simulink model "scheme"  (R2024a)
settings: Solver=VariableStepAuto  StartTime=0.0  StopTime=100  RelTol=1e-3
InitFcn:
  | A=[1 0; 1 1];
  | b=[3; 5];
  | d=b;
  | 
  | A0f=[0 1; -16 -8];
  | b0f=[0; 1];
  | N=b0f/d;
  | 
  | Ad=[0 1; -10.24 -6.4];
  | H=[1 0];
  | M=lyap(A,-Ad,-b*H);
  | K=H*inv(M);
  | Am=A-b*K;
  | Q=eye(2);
  | P=lyap(Am',Q);
settings Model: Creator=User  LastModifiedBy=alexe

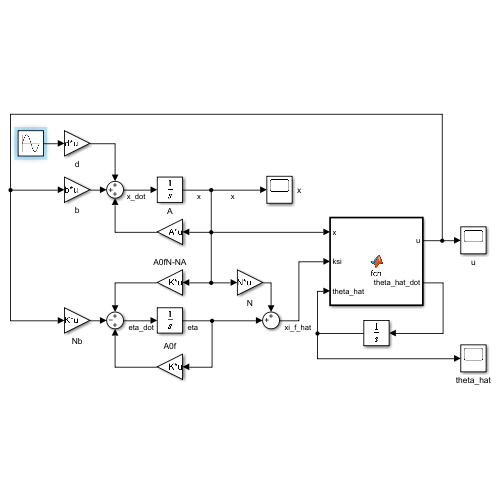
[thumbnail: Simulink's stored preview of the top-level diagram]
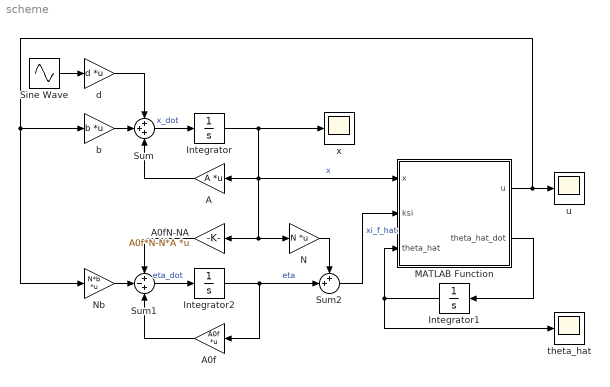
== system scheme ==
  A : Gain  Gain=A  Multiplication=Matrix(K*u)
  A0f : Gain  Gain=A0f  Multiplication=Matrix(K*u)
  A0fN-NA : Gain  Gain=A0f*N-N*A  Multiplication=Matrix(K*u)
  Integrator : Integrator  InitialCondition=[0; 0]
  Integrator1 : Integrator  InitialCondition=[0; 0]
  Integrator2 : Integrator  InitialCondition=[0; 0]
  MATLAB Function : MATLAB Function  TreatAsAtomicUnit=on
  N : Gain  Gain=N  Multiplication=Matrix(K*u)
  Nb : Gain  Gain=N*b  Multiplication=Matrix(K*u)
  Sine Wave : Sin  Amplitude=20  SampleTime=0
  Sum : Sum  Inputs=+++
  Sum1 : Sum  Inputs=+-+
  Sum2 : Sum  Inputs=++|
  b : Gain  Gain=b  Multiplication=Matrix(K*u)
  d : Gain  Gain=d  Multiplication=Matrix(K*u)
  theta_hat : Scope
  u : Scope
  x : Scope
  wires:
  Integrator/1 -> x/1, N/1, A0fN-NA/1, A/1, MATLAB Function/1(x)  "x"
  Sum/1 -> Integrator/1  "x_dot"
  MATLAB Function/2(theta_hat_dot) -> Integrator1/1
  MATLAB Function/1(u) -> u/1, Nb/1, b/1
  A/1 -> Sum/3
  b/1 -> Sum/2
  d/1 -> Sum/1
  Sine Wave/1 -> d/1
  Nb/1 -> Sum1/2
  A0f/1 -> Sum1/3
  Integrator2/1 -> A0f/1, Sum2/2  "eta"
  Sum1/1 -> Integrator2/1  "eta_dot"
  A0fN-NA/1 -> Sum1/1
  N/1 -> Sum2/1
  Sum2/1 -> MATLAB Function/2(ksi)  "xi_f_hat"
  Integrator1/1 -> theta_hat/1, MATLAB Function/3(theta_hat)

== matlab function scheme/MATLAB Function ==
  data: x input; ksi input; theta_hat input; u output; theta_hat_dot output; b parameter; P parameter; K parameter
function [u, theta_hat_dot] = fcn(x, ksi, theta_hat, b, P, K)
gamma=100;
u=-K*x-theta_hat'*ksi;
theta_hat_dot=gamma*ksi*b'*P*x;
